simulink model "acc_with_sensor"  (R2021b)
settings: Solver=FixedStepAuto  StartTime=0.0  StopTime=206  FixedStep=0.0005  RelTol=1e-3
InitFcn:
  | G=9.81;
  | m=1660;
  | rw=0.325;
  | Caf=74070;
  | Car=58525;
  | Iz=2778.5;
  | d = 1.502;
  | lf =1.1135;
  | lr =1.5065;
  | L = 2.62;
  | kph2mps=1/3.6;
values from neighbouring files (symbols this model uses):
  Leftdis_PV_switch = 2    [acc_plot_backup.m]
  s_path = [0 1.10508939428 2.2141958029 3.32141571172 4.42705301151 5.53154548532 6.63517443471 7.73808041313 8.84055018688 9.94289959674 11.0453539299 12.1480581097 ... (1001 elements, 1001x1)]    [200_100radius.mat]    (also in LV_Clothoid_S_Turn_path.mat = [0 0.966832089581 1.93621320584 2.90214024471 3.86476766313 ; NEDC_path.mat = [0 0.414605943146 0.832514087334 1.25401518562 1.68216660344; Straight_East_into_curve.mat = [0 1.65770560069 3.32192925577 4.98420060507 6.64484613518 8; acc_plot_backup.m = Station_HV_m)
  X_path = [0 1.10508939428 2.2141958029 3.32141571172 4.42705301151 5.53154548532 6.63517443471 7.73808041313 8.84055018688 9.94289959674 11.0453539299 12.1480581097 ... (1001 elements, 1001x1)]    [200_100radius.mat]    (also in LV_Clothoid_S_Turn_path.mat = [-10 -9.03316791042 -8.06378679416 -7.09785975529 -6.1352323; NEDC_path.mat = [0 0.414605943146 0.832514087334 1.25401518562 1.68216660344; Straight_East_into_curve.mat = [0 1.65770560069 3.32192925577 4.98420060507 6.64484613518 8; acc_plot_backup.m = X_HV_m)
  Y_path = [0 -1.70364610795e-18 -7.41532896709e-18 1.46822109542e-17 4.74557362791e-17 6.12980216762e-17 9.25043977736e-17 1.24088240159e-16 1.5099156923e-16 1.7058517853e-16 1.90629227614e-16 2.09673434424e-16 ... (1001 elements, 1001x1)]    [200_100radius.mat]    (also in LV_Clothoid_S_Turn_path.mat = [0 -8.46153035536e-19 5.07382551045e-18 2.07356032218e-17 3.; NEDC_path.mat = [0 -3.50680326162e-18 -2.14111304971e-18 3.38197671014e-18 3; Straight_East_into_curve.mat = [0 1.29197709199e-18 2.81882429322e-18 3.49020462564e-17 6.7; acc_plot_backup.m = Y_HV_m)
undefined symbols (not defined in the file or in its folder): C_TICK_TIME_S, Cut_in_Secenary_flg, ENUM_ACCSTATE_DISABLED, ENUM_ACCSTATE_OFF, ENUM_ACCSTATE_STANDBY, FALSE, KVDI_ACCLongPressTime_ms, KVDI_ACCMaxActSpeed_kph, KVDI_ACCSetSpdIntial_kph, KVDI_ACCSpdLargeChange_kph, KVDI_LongPressConTime_ms, ONE_FLOAT, ONE_INT, raptor_xcp_function, T, TRUE, UseTTC_switch, ZERO_FLOAT, ZERO_INT
libraries: ADASLibrary x29, simulink x22, Raptor_lib x11, dspstat3 x6, simulink_extras x6, Solver_SF x1, mpclib x1
(part 2 of 9)

== system acc_with_sensor/ACCSpdCalculation ==
  VDINR_VehSpd_kps : Inport
  NVDI_ACCActingPrev_flg : Inport  Port=2
  NVDI_ACCSystemStatePrev_enum : Inport  Port=3
  VDINR_ACCSpdSetDec_flg : Inport  Port=4
  VDINR_ACCSpdResInc_flg : Inport  Port=5
  Add : Sum  Inputs=+-
  Chart : Stateflow chart  TreatAsAtomicUnit=on
      settings: PortSchema="{\"entries\":[{\"content\":{\"sides\":[{\"content\":{\"connectorIds\":[\"In1\",\"In2\",\"In3\",\"In4\",\"In5\",\"In6\",\"In9\",\"In7\",\"In8\"]},\"type\":\"ConnectorPlacement.EquallySpacedRectSide\",\"uuid\":\"b1b09059-7c6b-4f2a-a509-9d89abb69bff\"},{\"content\":{\"connectorIds\":[\"Out2\",\"Out3\",\"Out1\"],\"side\":\"RIGHT\"},\"type\":\"ConnectorPlacement.EquallySpacedRectSide\",\"uuid\":\"426eb2b7-8f84-437e-9ce1-b8172d5a5373\"},{\"content\":{\"connectorIds\":[],\"side\":\"TOP\"},\"type\":\"ConnectorPlacement.EquallySpacedRectSide\",\"uuid\":\"808310a0-6f78-4728-b2e8-69880cb1a9d0\"}]},\"type\":\"ConnectorPlacement.EquallySpacedConnector\",\"uuid\":\"50fcbb31-1c9a-4815-926e-b0772552613f\"}],\"packageUris\":[\"http://schema.mathworks.com/mf0/Connector/R2020b\"],\"version\":\"1.0\"}"
  Constant : Constant  Value=KVDI_ACCLongPressTime_ms
  Constant1 : Constant  Value=KVDI_ACCSetSpdIntial_kph
  Constant2 : Constant  Value=KVDI_ACCSpdLargeChange_kph
  Constant3 : Constant  Value=ONE_FLOAT
  Constant4 : Constant  Value=KVDI_LongPressConTime_ms
  Delay : Delay  DelayLength=1
  Delay2 : Delay  DelayLength=1
  Divide : Product  Inputs=*/
  Equal : RelationalOperator  Operator===  OutDataTypeStr=boolean  RndMeth=Simplest
  KJUD_ACCMaxActSpeed_kph : Constant  Value=KVDI_ACCMaxActSpeed_kph
  Max : MinMax  Function=max  Inputs=2
  Max1 : MinMax  Inputs=2
  Max3 : MinMax  Function=max  Inputs=2
  Product : Product
  Round : Rounding  Operator=round
  Round1 : Rounding
  ZERO_FLOAT : Constant  Value=ZERO_FLOAT
  VVDI_ACCSetSpd_kph : Outport
  VVDI_ACCSpdInc_flg : Outport  Port=2
  VVDI_ACCSpdDec_flg : Outport  Port=3
  wires:
  Constant4/1 -> Chart/9(KVDI_LongPressConTime_ms)
  Chart/2(VVDI_ACCSpdInc_flg) -> VVDI_ACCSpdInc_flg/1
  Chart/3(VVDI_ACCSpdDec_flg) -> VVDI_ACCSpdDec_flg/1
  Max1/1 -> Max3/1
  KJUD_ACCMaxActSpeed_kph/1 -> Max1/2
  VDINR_ACCSpdSetDec_flg/1 -> Chart/2(VDINR_ACCSpdSetDec_flg), Delay/1, Add/1
  Constant3/1 -> Equal/2
  Delay/1 -> Add/2
  Add/1 -> Equal/1
  Equal/1 -> Chart/1(NVDI_SpdSet_flg)
  ZERO_FLOAT/1 -> Max3/2
  Chart/1(NVDI_ACCSetSpd_kph) -> Max1/1
  Product/1 -> Chart/8(NVDI_LongPressSpdIntial_kph)
  Divide/1 -> Round1/1
  Round1/1 -> Product/1
  Constant2/1 -> Divide/2, Product/2
  Delay2/1 -> Divide/1
  Round/1 -> Chart/4(NVDI_ACCSetSpdInitial_kph)
  VDINR_VehSpd_kps/1 -> Max/1  "VVDI_VehSpd_kph"
  Constant1/1 -> Max/2
  Max/1 -> Round/1
  NVDI_ACCSystemStatePrev_enum/1 -> Chart/6(NVDI_ACCSystemStatePrev_enum)
  NVDI_ACCActingPrev_flg/1 -> Chart/5(NVDI_ACCActingPrev_flg)
  Max3/1 -> VVDI_ACCSetSpd_kph/1, Delay2/1  "VVDI_ACCSetSpd_kph"
  VDINR_ACCSpdResInc_flg/1 -> Chart/3(VDINR_ACCSpdResInc_flg)
  Constant/1 -> Chart/7(KVDI_ACCLongPressTime_ms)

== system acc_with_sensor/ACC_Mode_Selector ==
  ACCSetSpeed_mps : Inport
  VACCTargetVehNotAssigned_flg : Inport  Port=2
  RR : Inport  Port=3
  Vx_HV_mps : Inport  Port=4
  RV : Inport  Port=5
  Add : Sum
  Add Constant : Bias  Bias=1
  Add13 : Sum  Inputs=-+
  Constant36 : Constant  Value=-0.5
  Logical Operator : Logic  Operator=OR  Inputs=3  AllPortsSameDT=off  OutDataTypeStr=boolean
  Logical Operator1 : Logic  AllPortsSameDT=off  OutDataTypeStr=boolean
  Logical Operator2 : Logic  Operator=NOT  AllPortsSameDT=off  OutDataTypeStr=boolean
  Logical Operator3 : Logic  AllPortsSameDT=off  OutDataTypeStr=boolean
  Relational Operator : RelationalOperator  Operator=<  OutDataTypeStr=boolean  RndMeth=Simplest
  Relational Operator1 : RelationalOperator  Operator=<  OutDataTypeStr=boolean  RndMeth=Simplest
  Relational Operator4 : RelationalOperator  Operator=<  OutDataTypeStr=boolean  RndMeth=Simplest
  Saturation : Saturate  UpperLimit=100  LowerLimit=0
  Saturation1 : Saturate  UpperLimit=100  LowerLimit=0
  Scope{,1..3,6..7,9..11} (9 alike) : Scope
  TH_ref : Gain  Gain=1.5
  TH_ref4 : Gain  Gain=1.5
  dist_safe1 : Bias  Bias=-2
  Out1 : Outport
  wires:
  Logical Operator/1 -> Out1/1, Scope11/1  "ACC_mode"
  [Vx_PV_mps] -> Add Constant/1
  VACCTargetVehNotAssigned_flg/1 -> Logical Operator2/1  "VACCTargetVehNotAssigned_flg"
  Relational Operator/1 -> Logical Operator1/1, Scope/1  "set_spd_compare"
  ACCSetSpeed_mps/1 -> [ACCSetSpeed_mps], Relational Operator/1
  Add/1 -> Saturation/1
  Vx_HV_mps/1 -> [Vx_HV_mps], Add/2
  RV/1 -> Add/1
  Saturation1/1 -> Add13/1, Relational Operator4/2  "act"
  TH_ref4/1 -> Scope3/1, Relational Operator4/1  "des"
  Relational Operator1/1 -> Logical Operator3/2, Scope7/1
  Constant36/1 -> Relational Operator1/2
  Add13/1 -> Scope10/1, Relational Operator1/1
  Logical Operator3/1 -> Scope1/1, Logical Operator/3  "dist_compare"
  TH_ref/1 -> Add13/2  "des"
  [ACCSetSpeed_mps] -> TH_ref4/1
  [Vx_HV_mps] -> TH_ref/1
  Relational Operator4/1 -> Logical Operator1/2, Scope6/1, Logical Operator3/1
  Saturation/1 -> [Vx_PV_mps]
  RR/1 -> dist_safe1/1
  Logical Operator1/1 -> Scope2/1, Logical Operator/2  "dist_compare"
  Add Constant/1 -> Relational Operator/2
  Logical Operator2/1 -> Scope9/1, [VACCTargetVehNotAssigned_flg], Logical Operator/1
  dist_safe1/1 -> Saturation1/1  "act"

== system acc_with_sensor/ACC_Mode_Selector3 ==
  ACCSetSpeed_mps : Inport
  VACCTargetVehNotAssigned_flg : Inport  Port=2
  RR : Inport  Port=3
  Vx_HV_mps : Inport  Port=4
  RV : Inport  Port=5
  Add : Sum
  Add1 : Sum  Inputs=-+
  Add2 : Sum  Inputs=+-
  Constant1 : Constant  Value=0.5
  Constant2 : Constant  Value=0.1
  Logical Operator : Logic  Operator=OR  AllPortsSameDT=off  OutDataTypeStr=boolean
  Logical Operator2 : Logic  Operator=NOT  AllPortsSameDT=off  OutDataTypeStr=boolean
  Logical Operator4 : Logic  Operator=NOT  Inputs=4  AllPortsSameDT=off  OutDataTypeStr=boolean
  Logical Operator5 : Logic  AllPortsSameDT=off  OutDataTypeStr=boolean
  Relational Operator5 : RelationalOperator  Operator=<  OutDataTypeStr=boolean  RndMeth=Simplest
  Relational Operator6 : RelationalOperator  Operator=<  OutDataTypeStr=boolean  RndMeth=Simplest
  Saturation : Saturate  UpperLimit=100  LowerLimit=0
  Saturation1 : Saturate  UpperLimit=100  LowerLimit=0
  Scope : Scope
  Scope1 : Scope
  TH_ref1 : Gain  Gain=1.5
  dist_safe1 : Bias  Bias=-2
  Out1 : Outport
  wires:
  dist_safe1/1 -> Saturation1/1  "act"
  Logical Operator2/1 -> Logical Operator/1
  RR/1 -> dist_safe1/1  "RR"
  Saturation/1 -> [Vx_PV_mps]
  Saturation1/1 -> Add1/2  "act_RR"
  RV/1 -> Add/1
  Vx_HV_mps/1 -> Add/2, [Vx_HV_mps]
  Add/1 -> Saturation/1
  VACCTargetVehNotAssigned_flg/1 -> Logical Operator2/1  "VACCTargetVehNotAssigned_flg"
  Logical Operator/1 -> Out1/1  "ACC_mode"
  Logical Operator5/1 -> Logical Operator4/1
  TH_ref1/1 -> Add1/1  "des"
  [Vx_HV_mps] -> TH_ref1/1
  Relational Operator6/1 -> Scope/1, Logical Operator5/2
  Add2/1 -> Relational Operator5/1
  Constant2/1 -> Relational Operator5/2
  Relational Operator5/1 -> Scope1/1, Logical Operator5/1  "set_spd_compare"
  Logical Operator4/1 -> Logical Operator/2  "ACC_mode"
  Add1/1 -> Relational Operator6/1
  Constant1/1 -> Relational Operator6/2
  ACCSetSpeed_mps/1 -> [ACCSetSpeed_mps]
  [Vx_PV_mps] -> Add2/1
  [ACCSetSpeed_mps] -> Add2/2

== system acc_with_sensor/Camera ==
  mps : Inport
  deg : Inport  Port=2
  Xo : Inport  Port=3
  Yo : Inport  Port=4
  station : Inport  Port=5
  Ax_HV_mps2 : Inport  Port=6
  Subsystem6 : Subsystem
  LeftDis : Outport
  wires:
  Subsystem6/1(LeftDis) -> LeftDis/1
  Ax_HV_mps2/1 -> Subsystem6/6(Ax_HV_mps2)
  deg/1 -> Subsystem6/2(deg)
  Yo/1 -> Subsystem6/4(Yo)
  Xo/1 -> Subsystem6/3(Xo)
  mps/1 -> Subsystem6/1(mps)
  station/1 -> Subsystem6/5(station)

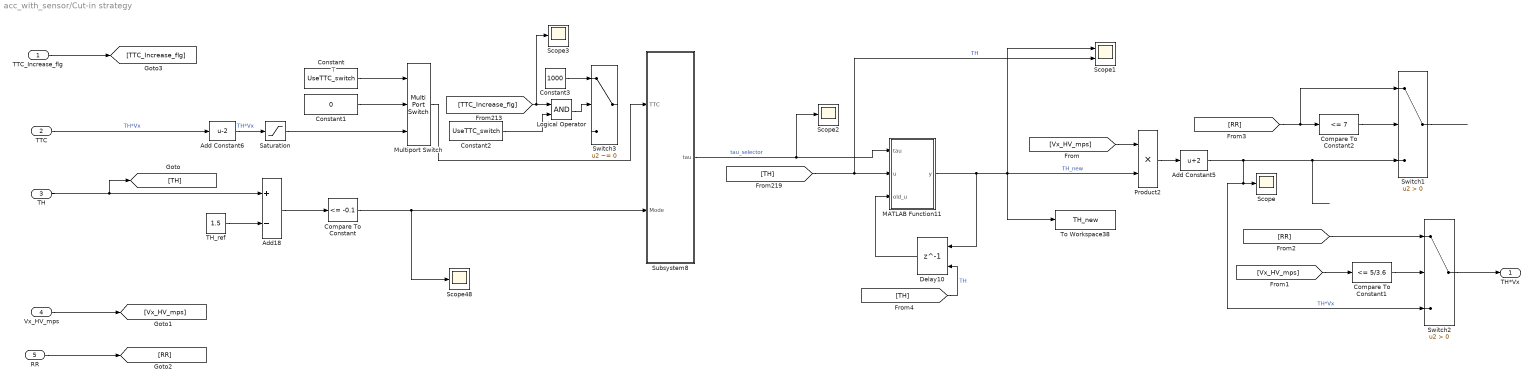
== system acc_with_sensor/Cut-in strategy ==
  note: T
  TTC_Increase_flg : Inport
  TTC : Inport  Port=2
  TH : Inport  Port=3
  Vx_HV_mps : Inport  Port=4
  RR : Inport  Port=5
  Add Constant5 : Bias  Bias=2
  Add Constant6 : Bias  Bias=-2
  Add18 : Sum  Inputs=+-
  Compare To Constant : simulink/Logic and Bit Operations/Compare To Constant  relop=<=  const=-0.1  OutDataTypeStr=boolean
  Compare To Constant1 : simulink/Logic and Bit Operations/Compare To Constant  relop=<=  const=5/3.6  OutDataTypeStr=boolean
  Compare To Constant2 : simulink/Logic and Bit Operations/Compare To Constant  relop=<=  const=7  OutDataTypeStr=boolean
  Constant : Constant  Value=UseTTC_switch  SampleTime=T
  Constant1 : Constant  Value=0  SampleTime=T
  Constant2 : Constant  Value=UseTTC_switch  SampleTime=T
  Constant3 : Constant  Value=1000
  Delay10 : Delay  DelayLength=1  InitialConditionSource=Input port  SampleTime=T
      settings: InputPortMap=u0,p4
  Logical Operator : Logic  AllPortsSameDT=off  OutDataTypeStr=boolean
  MATLAB Function11 : MATLAB Function  TreatAsAtomicUnit=on
  Multiport Switch : MultiPortSwitch  DataPortOrder=Zero-based contiguous  Inputs=2  zeroidx=on
  Product2 : Product
  Saturation : Saturate  UpperLimit=10  LowerLimit=0
  Scope{,2..3,48} (4 alike) : Scope
  Scope1 : Scope  NumInputPorts=2
  Subsystem8 : Subsystem
  Switch1 : Switch  Criteria=u2 > Threshold
  Switch2 : Switch  Criteria=u2 > Threshold
  Switch3 : Switch  Criteria=u2 ~= 0
  TH_ref : Constant  Value=1.5  SampleTime=T
  To Workspace38 : ToWorkspace  VariableName=TH_new  SampleTime=-1
  TH*Vx : Outport
  wires:
  [TH] -> Scope1/2, MATLAB Function11/2(u)  "TH"
  TH/1 -> Add18/1, [TH]
  Subsystem8/1(tau) -> Scope2/1, MATLAB Function11/1(tau)  "tau_selector"
  Add18/1 -> Compare To Constant/1
  MATLAB Function11/1(y) -> To Workspace38/1, Product2/2, Scope1/1, Delay10/1  "TH_new"
  TTC/1 -> Add Constant6/1  "TH*Vx"
  Delay10/1 -> MATLAB Function11/3(old_u)
  Product2/1 -> Add Constant5/1
  TH_ref/1 -> Add18/2
  Compare To Constant/1 -> Scope48/1, Subsystem8/2(Mode)
  Add Constant5/1 -> Switch2/3, Scope/1, Switch1/3  "TH*Vx"
  [Vx_HV_mps] -> Product2/1
  Vx_HV_mps/1 -> [Vx_HV_mps]
  RR/1 -> [RR]
  [RR] -> Switch1/1, Compare To Constant2/1
  Compare To Constant2/1 -> Switch1/2
  Switch1/1 -> ?
  [Vx_HV_mps] -> Compare To Constant1/1
  Compare To Constant1/1 -> Switch2/2
  [RR] -> Switch2/1
  Switch2/1 -> TH*Vx/1
  Saturation/1 -> Multiport Switch/3
  [TH] -> Delay10/2  "TH"
  Add Constant6/1 -> Saturation/1  "TH*Vx"
  Constant/1 -> Multiport Switch/1
  Constant1/1 -> Multiport Switch/2
  TTC_Increase_flg/1 -> [TTC_Increase_flg]
  [TTC_Increase_flg] -> Scope3/1, Logical Operator/1
  Constant3/1 -> Switch3/1
  Logical Operator/1 -> Switch3/2
  Multiport Switch/1 -> Subsystem8/1(TTC)
  Constant2/1 -> Logical Operator/2

== system acc_with_sensor/Latch ==
  set : Inport
  reset : Inport  Port=2
  Delay : Delay  DelayLength=1
  Logical Operator3 : Logic  AllPortsSameDT=off  OutDataTypeStr=boolean
  Logical Operator4 : Logic  Operator=NOT  AllPortsSameDT=off  OutDataTypeStr=boolean
  Switch : Switch  Criteria=u2 ~= 0
  Switch1 : Switch  Criteria=u2 ~= 0
  latched : Outport
  wires:
  Delay/1 -> Switch1/3
  Logical Operator4/1 -> Logical Operator3/2, Switch1/1
  Logical Operator3/1 -> Switch/2
  reset/1 -> Logical Operator4/1, Switch1/2
  Switch/1 -> Delay/1, latched/1
  set/1 -> Switch/1, Logical Operator3/1
  Switch1/1 -> Switch/3

== system acc_with_sensor/Latch2 ==
  set : Inport
  reset : Inport  Port=2
  Delay : Delay  DelayLength=1
  Logical Operator3 : Logic  AllPortsSameDT=off  OutDataTypeStr=boolean
  Logical Operator4 : Logic  Operator=NOT  AllPortsSameDT=off  OutDataTypeStr=boolean
  Switch : Switch  Criteria=u2 ~= 0
  Switch1 : Switch  Criteria=u2 ~= 0
  latched : Outport
  wires:
  Switch1/1 -> Switch/3
  set/1 -> Logical Operator3/1, Switch/1
  Switch/1 -> latched/1, Delay/1
  reset/1 -> Switch1/2, Logical Operator4/1
  Logical Operator3/1 -> Switch/2
  Logical Operator4/1 -> Switch1/1, Logical Operator3/2
  Delay/1 -> Switch1/3

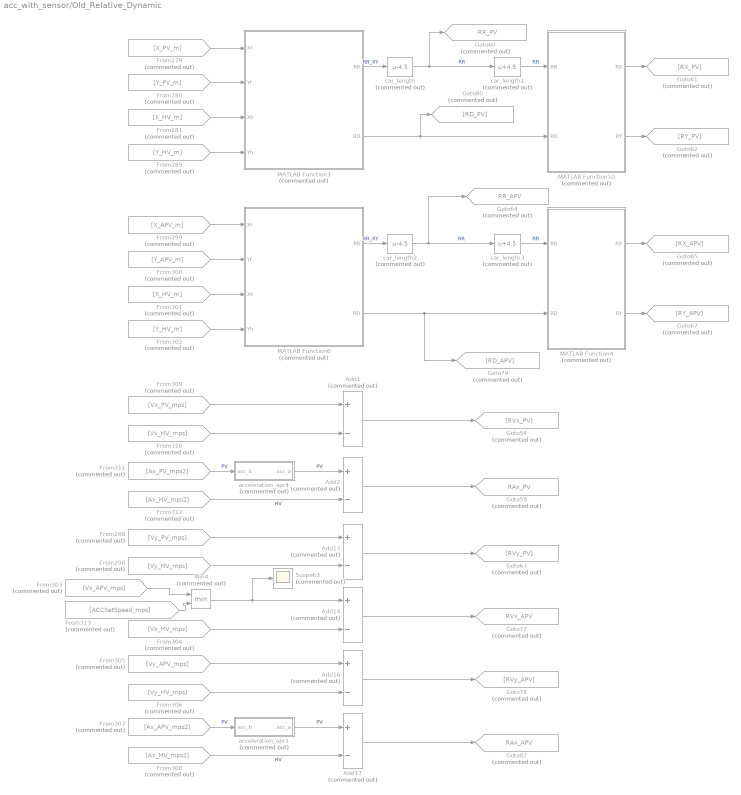
== system acc_with_sensor/Old_Relative_Dynamic ==
  Add{1..2,13..14,16..17} (6 alike) : Sum  Commented=on  Inputs=+-
  From279 : From  Commented=on  GotoTag=X_PV_m
  From280 : From  Commented=on  GotoTag=Y_PV_m
  From281 : From  Commented=on  GotoTag=X_HV_m
  From285 : From  Commented=on  GotoTag=Y_HV_m
  From288 : From  Commented=on  GotoTag=Vy_PV_mps
  From298 : From  Commented=on  GotoTag=Vy_HV_mps
  From299 : From  Commented=on  GotoTag=X_APV_m
  From300 : From  Commented=on  GotoTag=Y_APV_m
  From301 : From  Commented=on  GotoTag=X_HV_m
  From302 : From  Commented=on  GotoTag=Y_HV_m
  From303 : From  Commented=on  GotoTag=Vx_APV_mps
  From304 : From  Commented=on  GotoTag=Vx_HV_mps
  From305 : From  Commented=on  GotoTag=Vy_APV_mps
  From306 : From  Commented=on  GotoTag=Vy_HV_mps
  From307 : From  Commented=on  GotoTag=Ax_APV_mps2
  From308 : From  Commented=on  GotoTag=Ax_HV_mps2
  From309 : From  Commented=on  GotoTag=Vx_PV_mps
  From310 : From  Commented=on  GotoTag=Vx_HV_mps
  From311 : From  Commented=on  GotoTag=Ax_PV_mps2
  From312 : From  Commented=on  GotoTag=Ax_HV_mps2
  From313 : From  Commented=on  GotoTag=ACCSetSpeed_mps
  Goto54 : Goto  Commented=on  GotoTag=RVx_PV
  Goto59 : Goto  Commented=on  GotoTag=RAx_PV  TagVisibility=global
  Goto60 : Goto  Commented=on  GotoTag=RR_PV  TagVisibility=global
  Goto61 : Goto  Commented=on  GotoTag=RX_PV
  Goto62 : Goto  Commented=on  GotoTag=RY_PV
  Goto63 : Goto  Commented=on  GotoTag=RVy_PV
  Goto64 : Goto  Commented=on  GotoTag=RR_APV  TagVisibility=global
  Goto65 : Goto  Commented=on  GotoTag=RX_APV
  Goto67 : Goto  Commented=on  GotoTag=RY_APV
  Goto77 : Goto  Commented=on  GotoTag=RVx_APV  TagVisibility=global
  Goto78 : Goto  Commented=on  GotoTag=RVy_APV
  Goto79 : Goto  Commented=on  GotoTag=RD_APV
  Goto80 : Goto  Commented=on  GotoTag=RD_PV
  Goto82 : Goto  Commented=on  GotoTag=RAx_APV  TagVisibility=global
  MATLAB Function10 : MATLAB Function  Commented=on  TreatAsAtomicUnit=on
  MATLAB Function3 : MATLAB Function  Commented=on  TreatAsAtomicUnit=on
  MATLAB Function4 : MATLAB Function  Commented=on  TreatAsAtomicUnit=on
  MATLAB Function6 : MATLAB Function  Commented=on  TreatAsAtomicUnit=on
  Min4 : MinMax  Commented=on  Inputs=2
  Scope63 : Scope  Commented=on
  acceleration_apr1 : Subsystem  Commented=on
  acceleration_apr4 : Subsystem  Commented=on
  car_length : Bias  Commented=on  Bias=-4.5
  car_length1 : Bias  Commented=on  Bias=4.5
  car_length2 : Bias  Commented=on  Bias=-4.5
  car_length3 : Bias  Commented=on  Bias=4.5
  wires:
  acceleration_apr1/1(acc_a) -> Add17/1  "PV"
  From299/1 -> MATLAB Function6/1(Xf)
  Add2/1 -> Goto59/1
  MATLAB Function4/1(RX) -> Goto65/1
  From312/1 -> Add2/2  "HV"
  MATLAB Function6/2(RD) -> MATLAB Function4/2(RD), Goto79/1
  From303/1 -> Min4/1
  MATLAB Function3/1(RR) -> car_length/1  "RR_XY"
  From279/1 -> MATLAB Function3/1(Xf)
  Add16/1 -> Goto78/1
  car_length2/1 -> car_length3/1, Goto64/1  "RR"
  From285/1 -> MATLAB Function3/4(Yh)
  Add17/1 -> Goto82/1
  From301/1 -> MATLAB Function6/3(Xh)
  car_length1/1 -> MATLAB Function10/1(RR)  "RR"
  From300/1 -> MATLAB Function6/2(Yf)
  car_length/1 -> car_length1/1, Goto60/1  "RR"
  From309/1 -> Add1/1
  acceleration_apr4/1(acc_a) -> Add2/1  "PV"
  From281/1 -> MATLAB Function3/3(Xh)
  From288/1 -> Add13/1
  Add1/1 -> Goto54/1
  Add14/1 -> Goto77/1
  From280/1 -> MATLAB Function3/2(Yf)
  From298/1 -> Add13/2
  Min4/1 -> Scope63/1, Add14/1
  MATLAB Function10/2(RY) -> Goto62/1
  From305/1 -> Add16/1
  MATLAB Function10/1(RX) -> Goto61/1
  car_length3/1 -> MATLAB Function4/1(RR)  "RR"
  From306/1 -> Add16/2
  From310/1 -> Add1/2
  From304/1 -> Add14/2
  From313/1 -> Min4/2
  MATLAB Function6/1(RR) -> car_length2/1  "RR_XY"
  MATLAB Function3/2(RD) -> Goto80/1, MATLAB Function10/2(RD)
  From307/1 -> acceleration_apr1/1(acc_b)  "PV"
  From308/1 -> Add17/2  "HV"
  MATLAB Function4/2(RY) -> Goto67/1
  Add13/1 -> Goto63/1
  From302/1 -> MATLAB Function6/4(Yh)
  From311/1 -> acceleration_apr4/1(acc_b)  "PV"

== system acc_with_sensor/PV_trajectory_planning ==
  x_translate : Inport
  yaw_rotate : Inport  Port=2
  y_translate : Inport  Port=3
  Ry : Inport  Port=4
  Add61 : Sum
  Add64 : Sum
  Gain64 : Gain  Gain=-1
  Gain{65..68} (4 alike) : Gain  Gain=pi/180
  Product{3..6} (4 alike) : Product
  Scope{57,59,62..63} (4 alike) : Scope
  Sin1 : Trigonometry
  Sin2 : Trigonometry  Operator=cos
  Sin3 : Trigonometry  Operator=cos
  Sin4 : Trigonometry
  Switch7 : Switch
  Switch8 : Switch
  ascending1 : dspstat3/Sort  otype=Value  dir=Ascending  sortAlg=Quick sort  roundingMode=Floor  overflowMode=off  accumDataTypeStr=Inherit: Same as product output  accumLastDataTypeStr=Inherit: Same as product output
      settings: SourceProductBaseCode=DS
  descending1 : dspstat3/Sort  otype=Value  dir=Descending  sortAlg=Quick sort  roundingMode=Floor  overflowMode=off  accumDataTypeStr=Inherit: Same as product output  accumLastDataTypeStr=Inherit: Same as product output
      settings: SourceProductBaseCode=DS
  LeftDis_PV_multi : Outport
  wires:
  Add64/1 -> Scope59/1, Switch7/2
  Product5/1 -> Add64/1
  Gain68/1 -> Sin4/1
  Sin1/1 -> Gain64/1
  Gain64/1 -> Product3/2
  descending1/1 -> Switch8/3
  Ry/1 -> Scope62/1, Switch8/2, Switch7/3
  Sin4/1 -> Product6/2
  Gain67/1 -> Sin3/1
  Switch8/1 -> LeftDis_PV_multi/1
  [yaw_rotate] -> Gain68/1
  Sin3/1 -> Product5/2
  Product6/1 -> Add64/2
  Switch7/1 -> Scope57/1, ascending1/1, descending1/1
  Sin2/1 -> Product4/2
  Gain66/1 -> Sin2/1
  y_translate/1 -> [y_translate], Product4/1
  Gain65/1 -> Sin1/1
  [x_translate] -> Product5/1
  ascending1/1 -> Switch8/1
  Product4/1 -> Add61/2
  Add61/1 -> Scope63/1, Switch7/1
  Product3/1 -> Add61/1
  x_translate/1 -> Product3/1, [x_translate]
  [y_translate] -> Product6/1
  [yaw_rotate] -> Gain67/1
  yaw_rotate/1 -> [yaw_rotate], Gain65/1
  [yaw_rotate] -> Gain66/1

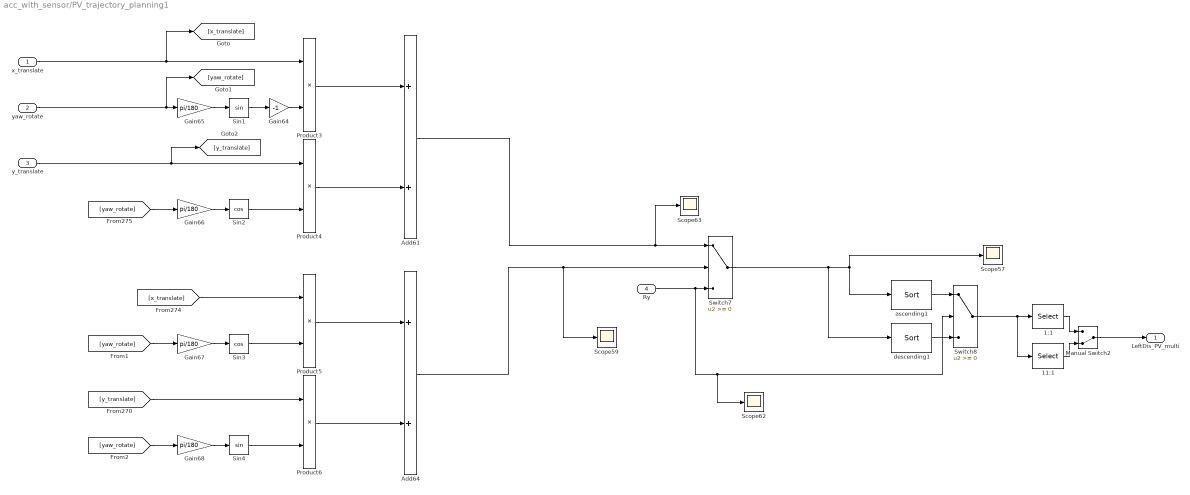
== system acc_with_sensor/PV_trajectory_planning1 ==
  x_translate : Inport
  yaw_rotate : Inport  Port=2
  y_translate : Inport  Port=3
  Ry : Inport  Port=4
  11:1 : Selector  InputPortWidth=20  IndexOptions=Index vector (dialog)  Indices=[11:20]  OutputSizes=1
  1:1 : Selector  InputPortWidth=20  IndexOptions=Index vector (dialog)  Indices=[1:10]  OutputSizes=1
  Add61 : Sum
  Add64 : Sum
  Gain64 : Gain  Gain=-1
  Gain{65..68} (4 alike) : Gain  Gain=pi/180
  Manual Switch2 : ManualSwitch  CurrentSetting=0
  Product{3..6} (4 alike) : Product
  Scope{57,59,62..63} (4 alike) : Scope
  Sin1 : Trigonometry
  Sin2 : Trigonometry  Operator=cos
  Sin3 : Trigonometry  Operator=cos
  Sin4 : Trigonometry
  Switch7 : Switch
  Switch8 : Switch
  ascending1 : dspstat3/Sort  otype=Value  dir=Ascending  sortAlg=Quick sort  roundingMode=Floor  overflowMode=off  accumDataTypeStr=Inherit: Same as product output  accumLastDataTypeStr=Inherit: Same as product output
      settings: SourceProductBaseCode=DS
  descending1 : dspstat3/Sort  otype=Value  dir=Descending  sortAlg=Quick sort  roundingMode=Floor  overflowMode=off  accumDataTypeStr=Inherit: Same as product output  accumLastDataTypeStr=Inherit: Same as product output
      settings: SourceProductBaseCode=DS
  LeftDis_PV_multi : Outport
  wires:
  Add64/1 -> Scope59/1, Switch7/2
  Product5/1 -> Add64/1
  Gain68/1 -> Sin4/1
  Sin1/1 -> Gain64/1
  Gain64/1 -> Product3/2
  descending1/1 -> Switch8/3
  Ry/1 -> Scope62/1, Switch8/2, Switch7/3
  Sin4/1 -> Product6/2
  Gain67/1 -> Sin3/1
  Switch8/1 -> 11:1/1, 1:1/1
  [yaw_rotate] -> Gain68/1
  Sin3/1 -> Product5/2
  Product6/1 -> Add64/2
  Switch7/1 -> Scope57/1, ascending1/1, descending1/1
  Sin2/1 -> Product4/2
  Gain66/1 -> Sin2/1
  y_translate/1 -> [y_translate], Product4/1
  Gain65/1 -> Sin1/1
  [x_translate] -> Product5/1
  ascending1/1 -> Switch8/1
  1:1/1 -> Manual Switch2/1
  Product4/1 -> Add61/2
  11:1/1 -> Manual Switch2/2
  Add61/1 -> Scope63/1, Switch7/1
  Product3/1 -> Add61/1
  Manual Switch2/1 -> LeftDis_PV_multi/1
  x_translate/1 -> Product3/1, [x_translate]
  [y_translate] -> Product6/1
  [yaw_rotate] -> Gain67/1
  yaw_rotate/1 -> [yaw_rotate], Gain65/1
  [yaw_rotate] -> Gain66/1

== system acc_with_sensor/R selector ==
  In1 : Inport
  vx : Inport  Port=2
  1-D Lookup Table2 : Lookup_n-D  NumberOfTableDimensions=1  BreakpointsForDimension1=[0 15 28 40]/3.6  Table=[31 31 35 35]  InternalRulePriority=Speed  RndMeth=Simplest  InputSameDT=on
  Constant1 : Constant  Value=35
  Constant19 : Constant
  Constant2 : Constant  Value=20
  Constant66 : Constant  Value=0.5
  Switch12 : Switch  Criteria=u2 > Threshold
  Out1 : Outport
  wires:
  Constant66/1 -> Switch12/1
  1-D Lookup Table2/1 -> Switch12/3
  In1/1 -> Switch12/2
  Switch12/1 -> Out1/1
  vx/1 -> 1-D Lookup Table2/1

== system acc_with_sensor/R selector1 ==
  In1 : Inport
  vx : Inport  Port=2
  1-D Lookup Table2 : Lookup_n-D  NumberOfTableDimensions=1  BreakpointsForDimension1=[0 15 28 40]/3.6  Table=[31 31 35 35]  InternalRulePriority=Speed  RndMeth=Simplest  InputSameDT=on
  Constant1 : Constant  Value=35
  Constant19 : Constant
  Constant2 : Constant  Value=7
  Constant66 : Constant  Value=0.5
  Switch12 : Switch  Criteria=u2 > Threshold
  Out1 : Outport
  wires:
  Switch12/1 -> Out1/1
  In1/1 -> Switch12/2
  Constant2/1 -> Switch12/3
  Constant66/1 -> Switch12/1

== system acc_with_sensor/R selector4 ==
  LaneAvail_fig : Inport
  vx : Inport  Port=2
  1-D Lookup Table2 : Lookup_n-D  NumberOfTableDimensions=1  BreakpointsForDimension1=[0 15 28 40]/3.6  Table=[31 31 35 35]  InternalRulePriority=Speed  RndMeth=Simplest  InputSameDT=on
  Constant1 : Constant  Value=35
  Constant19 : Constant
  Constant2 : Constant  Value=20
  Constant3 : Constant  Value=100
  Constant66 : Constant  Value=0.5  SampleTime=T
  Switch12 : Switch  Criteria=u2 > Threshold
  R : Outport
  wires:
  vx/1 -> 1-D Lookup Table2/1
  Switch12/1 -> R/1
  LaneAvail_fig/1 -> Switch12/2
  1-D Lookup Table2/1 -> Switch12/3
  Constant66/1 -> Switch12/1

== system acc_with_sensor/R selector5 ==
  LaneAvail_flg : Inport
  vx : Inport  Port=2
  1-D Lookup Table2 : Lookup_n-D  NumberOfTableDimensions=1  BreakpointsForDimension1=[0 15 28 40]/3.6  Table=[31 31 35 35]  InternalRulePriority=Speed  RndMeth=Simplest  InputSameDT=on
  Constant1 : Constant  Value=35
  Constant19 : Constant  Value=21
  Constant2 : Constant  Value=7
  Constant3 : Constant  Value=25
  Constant66 : Constant  Value=0.5
  Display : Display
  Switch12 : Switch  Criteria=u2 > Threshold
  R_D : Outport
  wires:
  Switch12/1 -> Display/1, R_D/1
  LaneAvail_flg/1 -> Switch12/2
  Constant2/1 -> Switch12/3
  Constant66/1 -> Switch12/1
  vx/1 -> 1-D Lookup Table2/1

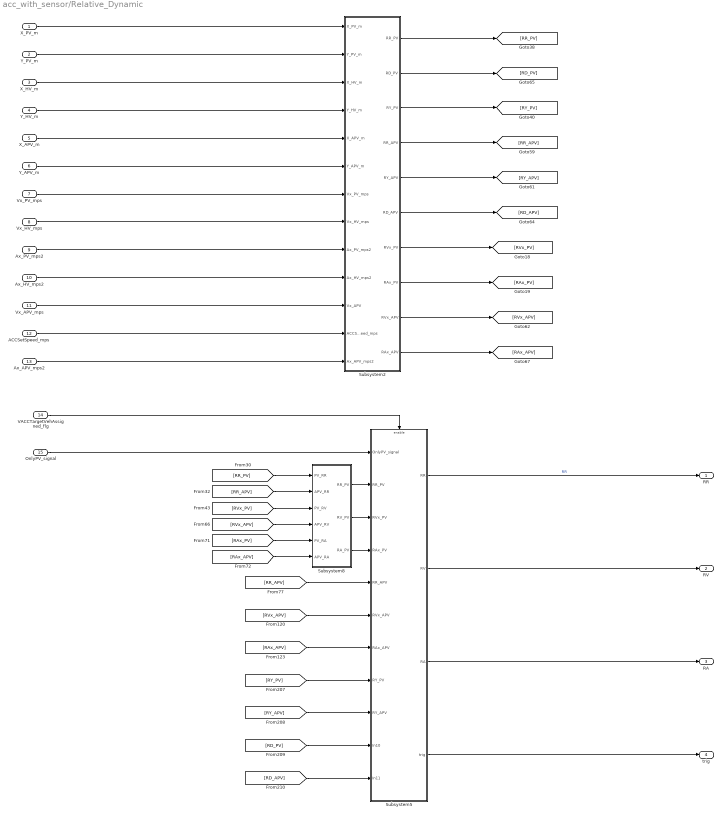
== system acc_with_sensor/Relative_Dynamic ==
  X_PV_m : Inport
  Y_PV_m : Inport  Port=2
  X_HV_m : Inport  Port=3
  Y_HV_m : Inport  Port=4
  X_APV_m : Inport  Port=5
  Y_APV_m : Inport  Port=6
  Vx_PV_mps : Inport  Port=7
  Vx_HV_mps : Inport  Port=8
  Ax_PV_mps2 : Inport  Port=9
  Ax_HV_mps2 : Inport  Port=10
  Vx_APV_mps : Inport  Port=11
  ACCSetSpeed_mps : Inport  Port=12
  Ax_APV_mps2 : Inport  Port=13
  VACCTargetVehAssigned_flg : Inport  Port=14
  OnlyPV_signal : Inport  Port=15
  Subsystem2 : Subsystem
  Subsystem5 : Subsystem
  Subsystem8 : Subsystem
  RR : Outport
  RV : Outport  Port=2
  RA : Outport  Port=3
  trig : Outport  Port=4
  wires:
  [RAx_APV] -> Subsystem8/6(APV_RA)
  [RAx_PV] -> Subsystem8/5(PV_RA)
  [RVx_APV] -> Subsystem8/4(APV_RV)
  [RVx_PV] -> Subsystem8/3(PV_RV)
  [RR_APV] -> Subsystem8/2(APV_RR)
  [RR_PV] -> Subsystem8/1(PV_RR)
  [RD_APV] -> Subsystem5/11(In11)
  [RD_PV] -> Subsystem5/10(In10)
  [RY_APV] -> Subsystem5/9(RY_APV)
  [RY_PV] -> Subsystem5/8(RY_PV)
  [RAx_APV] -> Subsystem5/7(RAx_APV)
  [RVx_APV] -> Subsystem5/6(RVx_APV)
  [RR_APV] -> Subsystem5/5(RR_APV)
  Subsystem2/6(RD_APV) -> [RD_APV]
  Subsystem8/1(RR_PV) -> Subsystem5/2(RR_PV)
  Subsystem2/4(RR_APV) -> [RR_APV]
  Y_APV_m/1 -> Subsystem2/6(Y_APV_m)
  Subsystem2/3(RY_PV) -> [RY_PV]
  ACCSetSpeed_mps/1 -> Subsystem2/12(ACCSetSpeed_mps)
  Y_PV_m/1 -> Subsystem2/2(Y_PV_m)
  Subsystem8/3(RA_PV) -> Subsystem5/4(RAx_PV)
  Subsystem8/2(RV_PV) -> Subsystem5/3(RVx_PV)
  Vx_HV_mps/1 -> Subsystem2/8(Vx_HV_mps)
  X_HV_m/1 -> Subsystem2/3(X_HV_m)
  Subsystem5/1(RR) -> RR/1  "RR"
  Subsystem2/1(RR_PV) -> [RR_PV]
  Subsystem2/7(RVx_PV) -> [RVx_PV]
  Y_HV_m/1 -> Subsystem2/4(Y_HV_m)
  Ax_PV_mps2/1 -> Subsystem2/9(Ax_PV_mps2)
  Subsystem2/8(RAx_PV) -> [RAx_PV]
  X_PV_m/1 -> Subsystem2/1(X_PV_m)
  Subsystem2/9(RVx_APV) -> [RVx_APV]
  OnlyPV_signal/1 -> Subsystem5/1(OnlyPV_signal)
  Subsystem2/5(RY_APV) -> [RY_APV]
  Subsystem2/2(RD_PV) -> [RD_PV]
  Subsystem2/10(RAx_APV) -> [RAx_APV]
  Vx_APV_mps/1 -> Subsystem2/11(Vx_APV)
  Ax_APV_mps2/1 -> Subsystem2/13(Ax_APV_mps2)
  X_APV_m/1 -> Subsystem2/5(X_APV_m)
  Vx_PV_mps/1 -> Subsystem2/7(Vx_PV_mps)
  VACCTargetVehAssigned_flg/1 -> Subsystem5/Enable
  Ax_HV_mps2/1 -> Subsystem2/10(Ax_HV_mps2)
  Subsystem5/2(RV) -> RV/1
  Subsystem5/3(RA) -> RA/1
  Subsystem5/4(trig) -> trig/1

== system acc_with_sensor/Smooth Switch ==
  Spd_acc_cmd : Inport
  Mode : Inport  Port=2
  TH_acc_cmd : Inport  Port=3
  TTC : Inport  Port=4
  Add12 : Sum
  Add9 : Sum  Inputs=+-
  Constant49 : Constant
  Data Type Conversion : DataTypeConversion  OutDataTypeStr=double
  Delay : Delay  DelayLength=1  InitialConditionSource=Input port  SampleTime=T
      settings: InputPortMap=u0,p4
  MATLAB Function : MATLAB Function  TreatAsAtomicUnit=on
  Product1 : Product
  Product2 : Product
  Scope : Scope
  Subsystem : Subsystem
  ax_cmd : Outport
  wires:
  Product2/1 -> Add12/1
  Spd_acc_cmd/1 -> Product2/1
  MATLAB Function/1(y) -> Delay/1, Scope/1, Add9/2, Product2/2
  Data Type Conversion/1 -> Delay/2, MATLAB Function/2(u)
  Constant49/1 -> Add9/1
  Product1/1 -> Add12/2
  TH_acc_cmd/1 -> Product1/2
  Add9/1 -> Product1/1
  Add12/1 -> ax_cmd/1
  Mode/1 -> Subsystem/2(Mode), Data Type Conversion/1
  Delay/1 -> MATLAB Function/3(old_u)
  Subsystem/1(tau) -> MATLAB Function/1(tau)  "tau_selector"
  TTC/1 -> Subsystem/1(TTC)

== system acc_with_sensor/Smooth Switch1 ==
  Dynamic_cmd : Inport
  Mode : Inport  Port=2
  Kinematic_cmd : Inport  Port=3
  Add12 : Sum
  Add9 : Sum  Inputs=+-
  Constant1 : Constant  Value=50
  Constant2 : Constant  Value=-50
  Constant49 : Constant
  Data Type Conversion : DataTypeConversion  OutDataTypeStr=double
  Product1 : Product
  Product2 : Product
  Rate Limiter : ADASLibrary/Rate Limiter  T=T
      settings: SourceProductName=ADASLibrary
  Scope : Scope  NumInputPorts=2
  Smooth_Switch1 : Subsystem  mask{tau=0.5, IC=0, T=T}
      mask prompts: tau "Time constant"; T "Sample time"
      mask Display:
      | fprintf('Discrete first order \n\n')
      | fprintf(['tau=' num2str(tau) '    IC=' num2str(IC)])
  ax_cmd : Outport
  wires:
  Mode/1 -> Data Type Conversion/1
  Add9/1 -> Product1/1
  Kinematic_cmd/1 -> Product1/2
  Product1/1 -> Add12/2
  Constant49/1 -> Add9/1
  Data Type Conversion/1 -> Product2/2, Add9/2
  Dynamic_cmd/1 -> Product2/1
  Product2/1 -> Add12/1
  Add12/1 -> Rate Limiter/2, ax_cmd/1, Scope/1
  Constant1/1 -> Rate Limiter/1
  Constant2/1 -> Rate Limiter/3
  Rate Limiter/1 -> Scope/2

== system acc_with_sensor/Smooth Switch4 ==
  Spd_acc_cmd : Inport
  Mode : Inport  Port=2
  TH_acc_cmd : Inport  Port=3
  Add12 : Sum
  Add9 : Sum  Inputs=+-
  Constant49 : Constant
  Data Type Conversion : DataTypeConversion  OutDataTypeStr=double
  Delay : Delay  DelayLength=1  InitialConditionSource=Input port  SampleTime=T
      settings: InputPortMap=u0,p4
  MATLAB Function : MATLAB Function  TreatAsAtomicUnit=on
  Product1 : Product
  Product2 : Product
  Scope : Scope
  Subsystem : Subsystem
  ax_cmd : Outport
  wires:
  Product2/1 -> Add12/1
  Spd_acc_cmd/1 -> Product2/1
  MATLAB Function/1(y) -> Delay/1, Scope/1, Add9/2, Product2/2
  Data Type Conversion/1 -> Delay/2, MATLAB Function/2(u)
  Constant49/1 -> Add9/1
  Product1/1 -> Add12/2
  TH_acc_cmd/1 -> Product1/2
  Add9/1 -> Product1/1
  Add12/1 -> ax_cmd/1
  Mode/1 -> Data Type Conversion/1
  Delay/1 -> MATLAB Function/3(old_u)
  Subsystem/1(tau) -> MATLAB Function/1(tau)  "tau_selector"

== system acc_with_sensor/Steer_Dynamic ==
  Model : Inport
  Q : Inport  Port=2
  R : Inport  Port=3
  u_old : Inport  Port=4
  Enable : EnablePort  StatesWhenEnabling=reset
  Bus Selector : BusSelector  OutputSignals=A,B,C,Yref,x_state
  Constant104 : Constant  Value=Np  SampleTime=T
  Constant105 : Constant  Value=Nc  SampleTime=T
  MPC_ACC4 : MATLAB Function  TreatAsAtomicUnit=on
  cmd : Outport
  wires:
  Constant105/1 -> MPC_ACC4/7(Nc)
  MPC_ACC4/1(u) -> cmd/1  "cmd"
  Q/1 -> MPC_ACC4/8(Qs)
  Constant104/1 -> MPC_ACC4/6(Np)
  R/1 -> MPC_ACC4/9(Rs)
  u_old/1 -> MPC_ACC4/10(u_old)
  Model/1 -> Bus Selector/1
  Bus Selector/1 -> MPC_ACC4/1(A)  "<A>"
  Bus Selector/2 -> MPC_ACC4/2(B)  "<B>"
  Bus Selector/3 -> MPC_ACC4/3(C)  "<C>"
  Bus Selector/4 -> MPC_ACC4/4(Yref)  "<Yref>"
  Bus Selector/5 -> MPC_ACC4/5(x_state)  "<x_state>"

== system acc_with_sensor/Steer_Kinematic ==
  Model : Inport
  Q : Inport  Port=2
  R : Inport  Port=3
  u_old : Inport  Port=4
  Enable : EnablePort  StatesWhenEnabling=reset
  Bus Selector : BusSelector  OutputSignals=A,B,C,Yref,x_state
  Constant104 : Constant  Value=Np  SampleTime=T
  Constant105 : Constant  Value=Nc  SampleTime=T
  MPC_ACC4 : MATLAB Function  TreatAsAtomicUnit=on
  cmd : Outport
  wires:
  u_old/1 -> MPC_ACC4/10(u_old)
  R/1 -> MPC_ACC4/9(Rs)
  Constant104/1 -> MPC_ACC4/6(Np)
  Q/1 -> MPC_ACC4/8(Qs)
  MPC_ACC4/1(u) -> cmd/1  "cmd"
  Constant105/1 -> MPC_ACC4/7(Nc)
  Model/1 -> Bus Selector/1
  Bus Selector/1 -> MPC_ACC4/1(A)  "<A>"
  Bus Selector/2 -> MPC_ACC4/2(B)  "<B>"
  Bus Selector/3 -> MPC_ACC4/3(C)  "<C>"
  Bus Selector/4 -> MPC_ACC4/4(Yref)  "<Yref>"
  Bus Selector/5 -> MPC_ACC4/5(x_state)  "<x_state>"

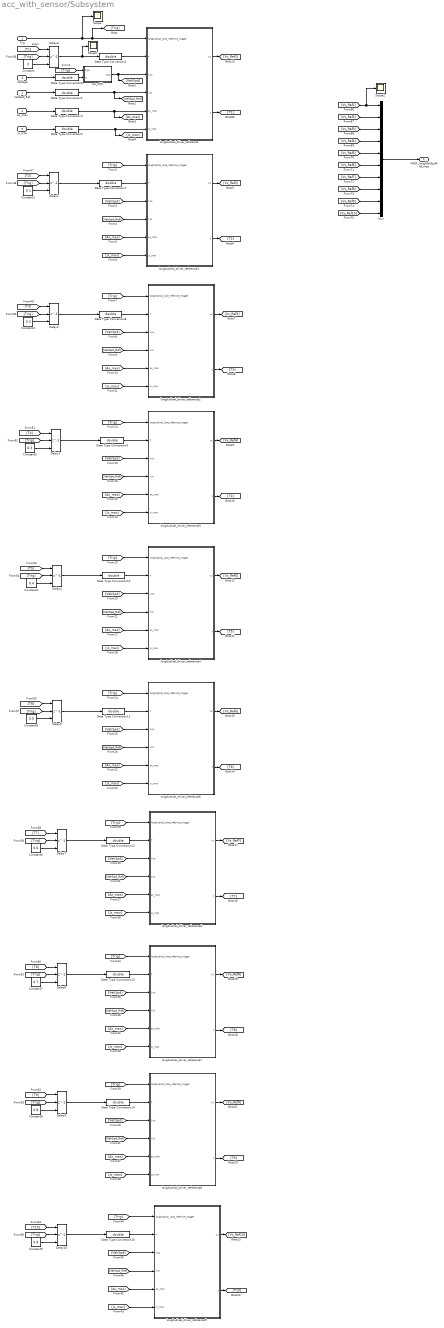
== system acc_with_sensor/Subsystem ==
  "Trig " : Inport
  VehSpd_Ref : Inport  Port=2
  VehSpd : Inport  Port=3
  Ax_max : Inport  Port=4
  Jx_max : Inport  Port=5
  Constant : Constant  Value=0
  Constant1 : Constant  Value=0.1  SampleTime=T
  Constant2 : Constant  Value=0.2
  Constant3 : Constant  Value=0.3
  Constant4 : Constant  Value=0.4
  Constant5 : Constant  Value=0.5
  Constant6 : Constant  Value=0.6
  Constant7 : Constant  Value=0.7
  Constant8 : Constant  Value=0.8
  Constant9 : Constant  Value=0.9
  Data Type Conversion{1..2,4..15} (14 alike) : DataTypeConversion  OutDataTypeStr=double
  Delay{1..10} (10 alike) : Delay  DelayLength=1  InitialConditionSource=Input port  ExternalReset=Rising
      settings: InputPortMap=u0,r5,p4
  Mux : Mux  Inputs=10
  Scope : Scope
  Scope1 : Scope
  Scope2 : Scope
  cut_off5 : Subsystem
  longitudinal_driver_reference : MATLAB Function  TreatAsAtomicUnit=on
  longitudinal_driver_reference1 : MATLAB Function  TreatAsAtomicUnit=on
  longitudinal_driver_reference2 : MATLAB Function  TreatAsAtomicUnit=on
  longitudinal_driver_reference3 : MATLAB Function  TreatAsAtomicUnit=on
  longitudinal_driver_reference4 : MATLAB Function  TreatAsAtomicUnit=on
  longitudinal_driver_reference5 : MATLAB Function  TreatAsAtomicUnit=on
  longitudinal_driver_reference6 : MATLAB Function  TreatAsAtomicUnit=on
  longitudinal_driver_reference7 : MATLAB Function  TreatAsAtomicUnit=on
  longitudinal_driver_reference8 : MATLAB Function  TreatAsAtomicUnit=on
  longitudinal_driver_reference9 : MATLAB Function  TreatAsAtomicUnit=on
  "VREF_LongiVehSpdRef_mps " : Outport
  wires:
  longitudinal_driver_reference/1(Vx) -> [Vx_Ref1]
  Mux/1 -> "VREF_LongiVehSpdRef_mps "/1
  Constant/1 -> Delay6/3
  [T1] -> Delay6/1
  Ax_max/1 -> Data Type Conversion4/1
  Jx_max/1 -> Data Type Conversion5/1
  VehSpd_Ref/1 -> Data Type Conversion1/1
  longitudinal_driver_reference/2(t) -> [T1]
  Delay6/1 -> Scope1/1, Data Type Conversion2/1
  [Trig] -> Delay6/2
  "Trig "/1 -> Scope/1, [Trig], longitudinal_driver_reference/1(longitudinal_lane_refernce_trigger)
  Data Type Conversion2/1 -> longitudinal_driver_reference/2(T)
  VehSpd/1 -> Data Type Conversion6/1
  Data Type Conversion1/1 -> [VehSpd_Ref], longitudinal_driver_reference/4(Vxt)
  cut_off5/1(Out) -> [VehSpd], longitudinal_driver_reference/3(Vxo)
  Data Type Conversion6/1 -> cut_off5/2(in)
  [Trig] -> cut_off5/1(sign)
  Data Type Conversion5/1 -> [Jx_max], longitudinal_driver_reference/6(jx_max)
  Data Type Conversion4/1 -> [Ax_max], longitudinal_driver_reference/5(ax_max)
  [Trig] -> longitudinal_driver_reference1/1(longitudinal_lane_refernce_trigger)
  [VehSpd] -> longitudinal_driver_reference1/3(Vxo)
  [VehSpd_Ref] -> longitudinal_driver_reference1/4(Vxt)
  [Ax_max] -> longitudinal_driver_reference1/5(ax_max)
  [Jx_max] -> longitudinal_driver_reference1/6(jx_max)
  [Jx_max] -> longitudinal_driver_reference2/6(jx_max)
  [Ax_max] -> longitudinal_driver_reference2/5(ax_max)
  [VehSpd_Ref] -> longitudinal_driver_reference2/4(Vxt)
  [VehSpd] -> longitudinal_driver_reference2/3(Vxo)
  [Trig] -> longitudinal_driver_reference2/1(longitudinal_lane_refernce_trigger)
  [Trig] -> longitudinal_driver_reference3/1(longitudinal_lane_refernce_trigger)
  [VehSpd] -> longitudinal_driver_reference3/3(Vxo)
  [VehSpd_Ref] -> longitudinal_driver_reference3/4(Vxt)
  [Ax_max] -> longitudinal_driver_reference3/5(ax_max)
  [Jx_max] -> longitudinal_driver_reference3/6(jx_max)
  [Jx_max] -> longitudinal_driver_reference4/6(jx_max)
  [Ax_max] -> longitudinal_driver_reference4/5(ax_max)
  [VehSpd_Ref] -> longitudinal_driver_reference4/4(Vxt)
  [VehSpd] -> longitudinal_driver_reference4/3(Vxo)
  [Trig] -> longitudinal_driver_reference4/1(longitudinal_lane_refernce_trigger)
  [Trig] -> longitudinal_driver_reference5/1(longitudinal_lane_refernce_trigger)
  [VehSpd] -> longitudinal_driver_reference5/3(Vxo)
  [VehSpd_Ref] -> longitudinal_driver_reference5/4(Vxt)
  [Ax_max] -> longitudinal_driver_reference5/5(ax_max)
  [Jx_max] -> longitudinal_driver_reference5/6(jx_max)
  [Jx_max] -> longitudinal_driver_reference6/6(jx_max)
  [Ax_max] -> longitudinal_driver_reference6/5(ax_max)
  [VehSpd_Ref] -> longitudinal_driver_reference6/4(Vxt)
  [VehSpd] -> longitudinal_driver_reference6/3(Vxo)
  [Trig] -> longitudinal_driver_reference6/1(longitudinal_lane_refernce_trigger)
  [Trig] -> longitudinal_driver_reference7/1(longitudinal_lane_refernce_trigger)
  [VehSpd] -> longitudinal_driver_reference7/3(Vxo)
  [VehSpd_Ref] -> longitudinal_driver_reference7/4(Vxt)
  [Ax_max] -> longitudinal_driver_reference7/5(ax_max)
  [Jx_max] -> longitudinal_driver_reference7/6(jx_max)
  [Jx_max] -> longitudinal_driver_reference8/6(jx_max)
  [Ax_max] -> longitudinal_driver_reference8/5(ax_max)
  [VehSpd_Ref] -> longitudinal_driver_reference8/4(Vxt)
  [VehSpd] -> longitudinal_driver_reference8/3(Vxo)
  [Trig] -> longitudinal_driver_reference8/1(longitudinal_lane_refernce_trigger)
  [Trig] -> longitudinal_driver_reference9/1(longitudinal_lane_refernce_trigger)
  [VehSpd] -> longitudinal_driver_reference9/3(Vxo)
  [VehSpd_Ref] -> longitudinal_driver_reference9/4(Vxt)
  [Ax_max] -> longitudinal_driver_reference9/5(ax_max)
  [Jx_max] -> longitudinal_driver_reference9/6(jx_max)
  longitudinal_driver_reference1/1(Vx) -> [Vx_Ref2]
  longitudinal_driver_reference1/2(t) -> [T2]
  [Trig] -> Delay1/2
  Delay1/1 -> Data Type Conversion7/1
  [T2] -> Delay1/1
  Data Type Conversion7/1 -> longitudinal_driver_reference1/2(T)
  Constant1/1 -> Delay1/3
  Constant2/1 -> Delay2/3
  Data Type Conversion8/1 -> longitudinal_driver_reference2/2(T)
  [T3] -> Delay2/1
  Delay2/1 -> Data Type Conversion8/1
  [Trig] -> Delay2/2
  longitudinal_driver_reference2/2(t) -> [T3]
  longitudinal_driver_reference2/1(Vx) -> [Vx_Ref3]
  [Trig] -> Delay3/2
  Delay3/1 -> Data Type Conversion9/1
  [T4] -> Delay3/1
  Data Type Conversion9/1 -> longitudinal_driver_reference3/2(T)
  Constant3/1 -> Delay3/3
  longitudinal_driver_reference3/1(Vx) -> [Vx_Ref4]
  longitudinal_driver_reference3/2(t) -> [T4]
  Constant4/1 -> Delay4/3
  Data Type Conversion10/1 -> longitudinal_driver_reference4/2(T)
  [T5] -> Delay4/1
  Delay4/1 -> Data Type Conversion10/1
  [Trig] -> Delay4/2
  longitudinal_driver_reference4/2(t) -> [T5]
  longitudinal_driver_reference4/1(Vx) -> [Vx_Ref5]
  longitudinal_driver_reference5/1(Vx) -> [Vx_Ref6]
  longitudinal_driver_reference5/2(t) -> [T6]
  [Trig] -> Delay5/2
  Delay5/1 -> Data Type Conversion11/1
  [T6] -> Delay5/1
  Constant5/1 -> Delay5/3
  Data Type Conversion11/1 -> longitudinal_driver_reference5/2(T)
  longitudinal_driver_reference6/2(t) -> [T7]
  longitudinal_driver_reference6/1(Vx) -> [Vx_Ref7]
  Constant6/1 -> Delay7/3
  [T7] -> Delay7/1
  Delay7/1 -> Data Type Conversion12/1
  [Trig] -> Delay7/2
  Data Type Conversion12/1 -> longitudinal_driver_reference6/2(T)
  [Trig] -> Delay8/2
  Delay8/1 -> Data Type Conversion13/1
  [T8] -> Delay8/1
  Constant7/1 -> Delay8/3
  Data Type Conversion13/1 -> longitudinal_driver_reference7/2(T)
  longitudinal_driver_reference7/1(Vx) -> [Vx_Ref8]
  longitudinal_driver_reference7/2(t) -> [T8]
  longitudinal_driver_reference8/2(t) -> [T9]
  longitudinal_driver_reference8/1(Vx) -> [Vx_Ref9]
  Data Type Conversion14/1 -> longitudinal_driver_reference8/2(T)
  Constant8/1 -> Delay9/3
  [T9] -> Delay9/1
  Delay9/1 -> Data Type Conversion14/1
  [Trig] -> Delay9/2
  longitudinal_driver_reference9/1(Vx) -> [Vx_Ref10]
  longitudinal_driver_reference9/2(t) -> [T10]
  [Trig] -> Delay10/2
  Delay10/1 -> Data Type Conversion15/1
  [T10] -> Delay10/1
  Constant9/1 -> Delay10/3
  Data Type Conversion15/1 -> longitudinal_driver_reference9/2(T)
  [Vx_Ref1] -> Scope2/1, Mux/1
  [Vx_Ref2] -> Mux/2
  [Vx_Ref3] -> Mux/3
  [Vx_Ref4] -> Mux/4
  [Vx_Ref5] -> Mux/5
  [Vx_Ref6] -> Mux/6
  [Vx_Ref7] -> Mux/7
  [Vx_Ref8] -> Mux/8
  [Vx_Ref9] -> Mux/9
  [Vx_Ref10] -> Mux/10

== system acc_with_sensor/Subsystem1 ==
  In1 : Inport
  Constant117 : Constant  Value=single(1)  OutDataTypeStr=single
  Relational Operator : RelationalOperator  OutDataTypeStr=boolean  RndMeth=Simplest
  Saturation5 : Saturate  UpperLimit=inf  LowerLimit=40/3.6
  Switch7 : Switch  Criteria=u2 ~= 0
  Out1 : Outport
  wires:
  Relational Operator/1 -> Switch7/2
  In1/1 -> Relational Operator/1, Switch7/1
  Constant117/1 -> Relational Operator/2, Switch7/3
  Switch7/1 -> Out1/1

== system acc_with_sensor/Subsystem17 ==
  new_value : Inport
  Constant83 : Constant  Value=0.3
  Constant84 : Constant  Value=0.1
  Delay11 : Delay  DelayLength=1  SampleTime=T
  rolling_avg1 : Subsystem
  new_ave : Outport
  wires:
  new_value/1 -> rolling_avg1/1(new_value)
  rolling_avg1/1(new_ave) -> new_ave/1, Delay11/1
  Constant83/1 -> rolling_avg1/4(tc)
  Constant84/1 -> rolling_avg1/3(delta_t)  "T"
  Delay11/1 -> rolling_avg1/2(old_ave)

== system acc_with_sensor/Subsystem2 ==
  T_cmd : Inport
  Gain : Gain  Gain=-0.25
  Gain2 : Gain  Gain=1/250
  Gain3 : Gain  Gain=1/150
  Saturation1 : Saturate  UpperLimit=0  LowerLimit=-inf
  Smooth_Switch1 : Subsystem  mask{tau=0.3, IC=0, T=T}
      mask prompts: tau "Time constant"; T "Sample time"
      mask Display:
      | fprintf('Discrete first order \n\n')
      | fprintf(['tau=' num2str(tau) '    IC=' num2str(IC)])
  Smooth_Switch2 : Subsystem  mask{tau=0.3, IC=0, T=T}
      mask prompts: tau "Time constant"; T "Sample time"
      mask Display:
      | fprintf('Discrete first order \n\n')
      | fprintf(['tau=' num2str(tau) '    IC=' num2str(IC)])
  Subsystem : Subsystem
  Subsystem1 : Subsystem
  Transfer Fcn1 : TransferFcn  Denominator=[0.3 1]
  Transfer Fcn2 : TransferFcn  Denominator=[0.3 1]
  Pb_LF : Outport
  Pb_RF : Outport  Port=2
  Pb_RL : Outport  Port=3
  Pb_RR : Outport  Port=4
  wires:
  Subsystem1/1(new_ave) -> Pb_RL/1, Pb_RR/1
  Subsystem/1(new_ave) -> Pb_LF/1, Pb_RF/1
  Gain/1 -> Gain2/1, Gain3/1
  Saturation1/1 -> Gain/1
  T_cmd/1 -> Saturation1/1
  Gain2/1 -> Subsystem/1(new_value)
  Gain3/1 -> Subsystem1/1(new_value)

== system acc_with_sensor/Subsystem21 ==
  A : Inport
  B : Inport  Port=2
  C : Inport  Port=3
  Yref : Inport  Port=4
  x_state : Inport  Port=5
  u_old : Inport  Port=6
  Enable : EnablePort  StatesWhenEnabling=reset
  Constant104 : Constant  Value=Np  SampleTime=T
  Constant105 : Constant  Value=Nc  SampleTime=T
  Constant106 : Constant  Value=Q  SampleTime=T
  Constant107 : Constant  Value=R  SampleTime=T
  MPC_ACC4 : MATLAB Function  TreatAsAtomicUnit=on
  cmd : Outport
  wires:
  Constant107/1 -> MPC_ACC4/9(Rs)
  Constant104/1 -> MPC_ACC4/6(Np)
  Constant106/1 -> MPC_ACC4/8(Qs)
  MPC_ACC4/1(u) -> cmd/1  "cmd"
  Constant105/1 -> MPC_ACC4/7(Nc)
  A/1 -> MPC_ACC4/1(A)
  C/1 -> MPC_ACC4/3(C)
  Yref/1 -> MPC_ACC4/4(Yref)
  B/1 -> MPC_ACC4/2(B)
  x_state/1 -> MPC_ACC4/5(x_state)
  u_old/1 -> MPC_ACC4/10(u_old)

== system acc_with_sensor/Subsystem22 ==
  Est_switch : Inport
  RR_new : Inport  Port=2
  RVx : Inport  Port=3
  RAx : Inport  Port=4
  RR_est : Inport  Port=5
  RV_est : Inport  Port=6
  RA_est : Inport  Port=7
  ACCSetSpeed_mps : Inport  Port=8
  Vx_HV_mps : Inport  Port=9
  Ax_HV_mps2 : Inport  Port=10
  TH_trig : Inport  Port=11
  vx_p : Inport  Port=12
  Constant : Constant  SampleTime=T
  Constant1 : Constant  Value=0.1  SampleTime=T
  Constant2 : Constant  SampleTime=T
  Constant3 : Constant  Value=0.2  SampleTime=T
  Demux3 : Demux  Outputs=3
  MPC_TH : MATLAB Function  TreatAsAtomicUnit=on
  Multiport Switch2 : MultiPortSwitch  DataPortOrder=Zero-based contiguous  Inputs=2  DiagnosticForDefault=None  zeroidx=on
  Mux6 : Mux  Inputs=3
  Mux7 : Mux  Inputs=3
  Scope : Scope  NumInputPorts=2
  Scope1 : Scope
  Subsystem : Subsystem
  cmd_limiter1 : Subsystem
  cmd_limiter2 : Subsystem
  raptor_measurement : Raptor_lib/Data Storage/raptor_measurement  paramName='TH_acc'  nameSource=Parameter  calDispType=Number  calEnum={'False', 'True'}  calGain=1.0  calOffset=0.0  calMax=inf  calMin=-inf  calFormat='-1'  calUnit=''  calHelp=''  calAccess=1  calFunction=raptor_xcp_function(gcb)  calVisible=on
      settings: SourceProductName=Raptor
  raptor_measurement1 : Raptor_lib/Data Storage/raptor_measurement  paramName='Desired_distance'  nameSource=Parameter  calDispType=Number  calEnum={'False', 'True'}  calGain=1.0  calOffset=0.0  calMax=inf  calMin=-inf  calFormat='-1'  calUnit=''  calHelp=''  calAccess=1  calFunction=raptor_xcp_function(gcb)  calVisible=on
      settings: SourceProductName=Raptor
  th_acc : Outport
  Desired_distance : Outport  Port=2
  spd_acc : Outport  Port=3
  wires:
  Demux3/3 -> MPC_TH/6(ax_rel)  "Drel"
  Demux3/2 -> MPC_TH/5(V_rel)  "Drel"
  ACCSetSpeed_mps/1 -> MPC_TH/12(ACCSetSpeed_mps)
  cmd_limiter2/1(ax_cmd1) -> Scope/2, th_acc/1
  Est_switch/1 -> Multiport Switch2/1
  RA_est/1 -> Mux6/3
  RVx/1 -> Mux7/2
  Constant/1 -> MPC_TH/7(Qs_th)
  Vx_HV_mps/1 -> MPC_TH/2(vx_th)
  MPC_TH/2(Y_th) -> raptor_measurement1/1, Desired_distance/1
  Mux6/1 -> Multiport Switch2/3
  Mux7/1 -> Multiport Switch2/2
  Ax_HV_mps2/1 -> MPC_TH/3(ax_th)
  RAx/1 -> Mux7/3
  RR_est/1 -> Mux6/1
  Constant1/1 -> MPC_TH/8(Rs_th)
  Demux3/1 -> MPC_TH/4(D_rel)  "Drel"
  TH_trig/1 -> MPC_TH/1(long_trig)
  RR_new/1 -> Mux7/1
  RV_est/1 -> Mux6/2
  MPC_TH/1(u_TH) -> Scope/1, raptor_measurement/1, cmd_limiter2/1(ax_cmd)  "cmd"
  Multiport Switch2/1 -> Demux3/1, Scope1/1
  Constant2/1 -> MPC_TH/9(Qs_acc)
  Constant3/1 -> MPC_TH/10(Rs_acc)
  MPC_TH/3(u_acc) -> cmd_limiter1/1(ax_cmd)
  cmd_limiter1/1(ax_cmd1) -> spd_acc/1
  vx_p/1 -> MPC_TH/11(vx_p)

== system acc_with_sensor/Subsystem23 ==
  A : Inport
  B : Inport  Port=2
  C : Inport  Port=3
  Yref : Inport  Port=4
  x_state : Inport  Port=5
  u_old : Inport  Port=6
  Enable : EnablePort  StatesWhenEnabling=reset
  Constant104 : Constant  Value=Np  SampleTime=T
  Constant105 : Constant  Value=Nc  SampleTime=T
  Constant106 : Constant  Value=Q  SampleTime=T
  Constant107 : Constant  Value=R  SampleTime=T
  MPC_ACC4 : MATLAB Function  TreatAsAtomicUnit=on
  cmd : Outport
  wires:
  x_state/1 -> MPC_ACC4/5(x_state)
  B/1 -> MPC_ACC4/2(B)
  Yref/1 -> MPC_ACC4/4(Yref)
  C/1 -> MPC_ACC4/3(C)
  A/1 -> MPC_ACC4/1(A)
  Constant105/1 -> MPC_ACC4/7(Nc)
  MPC_ACC4/1(u) -> cmd/1  "cmd"
  Constant106/1 -> MPC_ACC4/8(Qs)
  Constant104/1 -> MPC_ACC4/6(Np)
  Constant107/1 -> MPC_ACC4/9(Rs)
  u_old/1 -> MPC_ACC4/10(u_old)

== system acc_with_sensor/Subsystem25 ==
  carsim : Inport
  Gain2 : Gain  Gain=pi/180
  Gain3 : Gain  Gain=1/20
  rad : Outport
  wires:
  Gain3/1 -> Gain2/1  "deg"
  Gain2/1 -> rad/1
  carsim/1 -> Gain3/1

== system acc_with_sensor/Subsystem3 ==
  Jerk : Inport
  Vx : Inport  Port=2
  Constant1 : Constant  Value=0  OutDataTypeStr=single  SampleTime=T
  Constant117 : Constant  Value=0.5  OutDataTypeStr=single  SampleTime=T
  Relational Operator : RelationalOperator  OutDataTypeStr=boolean  RndMeth=Simplest
  Switch7 : Switch  Criteria=u2 ~= 0
  Out1 : Outport
  wires:
  Relational Operator/1 -> Switch7/2
  Vx/1 -> Relational Operator/1
  Constant117/1 -> Relational Operator/2
  Switch7/1 -> Out1/1
  Constant1/1 -> Switch7/3
  Jerk/1 -> Switch7/1

== system acc_with_sensor/Subsystem4 ==
  new_value : Inport
  Constant44 : Constant  Value=0.25  SampleTime=T
  Constant48 : Constant  Value=0.1  SampleTime=T
  Delay1 : Delay  DelayLength=1  SampleTime=T
  rolling_avg1 : Subsystem
  new_ave : Outport
  wires:
  Constant44/1 -> rolling_avg1/4(tc)
  new_value/1 -> rolling_avg1/1(new_value)
  Constant48/1 -> rolling_avg1/3(delta_t)  "T"
  Delay1/1 -> rolling_avg1/2(old_ave)
  rolling_avg1/1(new_ave) -> new_ave/1, Delay1/1
